simulink model "Quadcopter_2D_Control"  (R2025a)
settings: Solver=VariableStepAuto  StartTime=0.0  StopTime=10.0  RelTol=1e-3
libraries: slpidlib x3
settings Model: Creator=TAKSH MEHTA  LastModifiedBy=TAKSH MEHTA

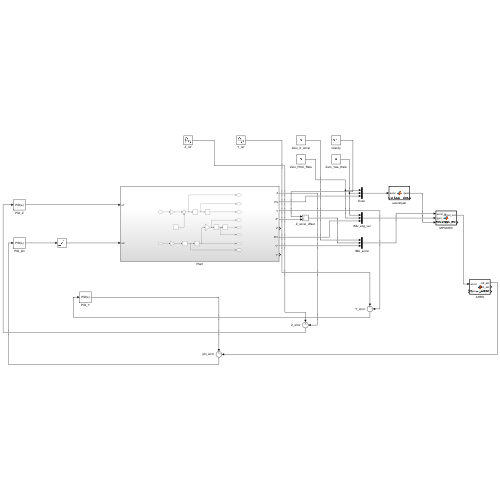
[thumbnail: Simulink's stored preview of the top-level diagram]
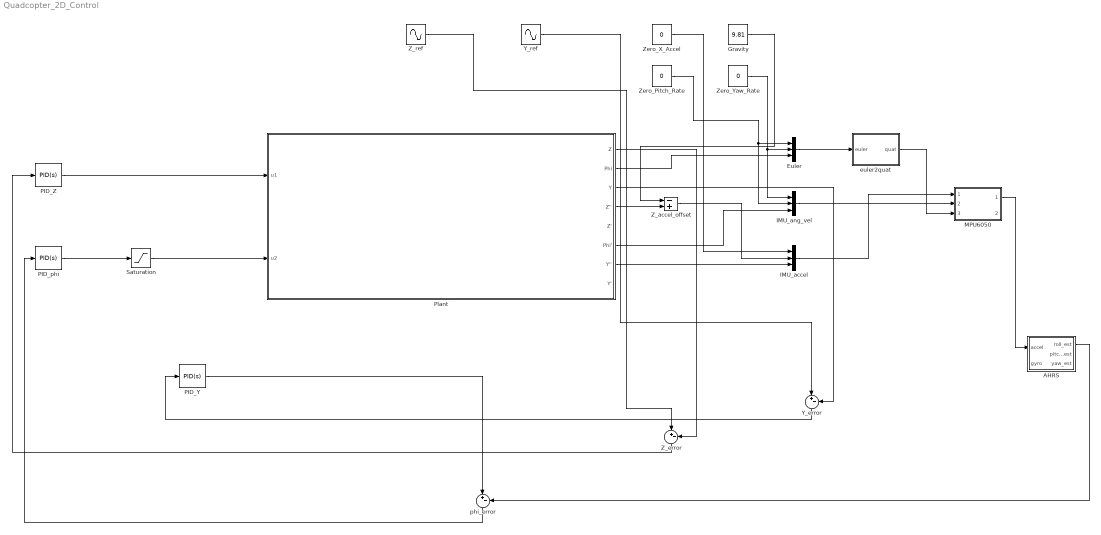
== system Quadcopter_2D_Control ==
  AHRS : MATLAB Function  TreatAsAtomicUnit=on
  Euler : Mux  Inputs=3
  Gravity : Constant  Value=9.81
  IMU_accel : Mux  Inputs=3
  IMU_ang_vel : Mux  Inputs=3
  MPU6050 : MATLAB Function  TreatAsAtomicUnit=on
  PID_Y : slpidlib/PID Controller  Controller=PID  Form=Parallel  TimeDomain=Continuous-time  UseExternalTs=off  SampleTime=-1  IntegratorMethod=Forward Euler  FilterMethod=Forward Euler  ControllerParametersSource=internal  P=2.2  I=0  UseKiTs=off  D=10  UseExternalDerivativeSource=off  N=100  UseFilter=on  TunerSelectOption=Transfer Function Based (PID Tuner App)  InitialConditionSource=internal  InitialConditionForIntegrator=0  InitialConditionForFilter=0  DifferentiatorICPrevScaledInput=0  ExternalReset=none  TrackingMode=off  Kt=1  LimitOutput=off  SatLimitsSource=internal  UpperSaturationLimit=inf  LowerSaturationLimit=-inf  LinearizeAsGain=on  AntiWindupMode=none  Kb=1  LimitIntegrator=off  UpperIntegratorSaturationLimit=inf  LowerIntegratorSaturationLimit=-inf  POutMin=[]  POutMax=[]  IOutMin=[]  IOutMax=[]  DOutMin=[]  DOutMax=[]  NOutMin=[]  NOutMax=[]  SumOutMin=[]  SumOutMax=[]  SaturationOutMin=[]  SaturationOutMax=[]  PParamMin=[]  PParamMax=[]  IParamMin=[]  IParamMax=[]  DParamMin=[]  DParamMax=[]  NParamMin=[]  NParamMax=[]  KbParamMin=[]  KbParamMax=[]  KtParamMin=[]  KtParamMax=[]  KbOutMin=[]  KbOutMax=[]  KtOutMin=[]  KtOutMax=[]  IntegratorOutMin=[]  IntegratorOutMax=[]  FilterOutMin=[]  FilterOutMax=[]  SumI1OutMin=[]  SumI1OutMax=[]  SumI2OutMin=[]  SumI2OutMax=[]  SumI3OutMin=[]  SumI3OutMax=[]  SumI4OutMin=[]  SumI4OutMax=[]  SumDOutMin=[]  SumDOutMax=[]  DifferentiatorOutMin=[]  DifferentiatorOutMax=[]  FilterDiffOutCoefMin=[]  FilterDiffOutCoefMax=[]  ReciprocalOutMin=[]  ReciprocalOutMax=[]  SumDenOutMin=[]  SumDenOutMax=[]  SumNumOutMin=[]  SumNumOutMax=[]  DivideOutMin=[]  DivideOutMax=[]  UdiffTsProdOutMin=[]  UdiffTsProdOutMax=[]  NTsProdOutMin=[]  NTsProdOutMax=[]  UintegralTsProdOutMin=[]  UintegralTsProdOutMax=[]  UngainTsProdOutMin=[]  UngainTsProdOutMax=[]  ClampingZeroOutDataTypeStr=Inherit: Inherit via back propagation  ClampingZeroOutMin=[]  ClampingZeroOutMax=[]  FilterDenConstantOutDataTypeStr=Inherit: Inherit via back propagation  FilterDenConstantOutMin=[]  FilterDenConstantOutMax=[]  PCopyOutDataTypeStr=Inherit: Inherit via back propagation  PCopyOutMin=[]  PCopyOutMax=[]  NCopyOutDataTypeStr=Inherit: Inherit via back propagation  NCopyOutMin=[]  NCopyOutMax=[]  IntegratorContinuousStateAttributes=''  IntegratorStateMustResolveToSignalObject=off  IntegratorRTWStateStorageClass=Auto  FilterContinuousStateAttributes=''  FilterStateMustResolveToSignalObject=off  FilterRTWStateStorageClass=Auto  ParallelPVariant=InternalParameters  IdealPVariant=Disabled  IVariant=InternalParameters  DVariant=InternalParameters  IntegratorVariant=Continuous  SatVariant=Disabled  AWVariant=Passthrough  PCopyVariant=Disabled  TRVariant=Disabled  FdbkBlocksVariant=Forward  IdealPFdbkVariant=Disabled  SatFdbkVariant=Disabled  DerivativeFilterVariant=ContFilter  NVariant=InternalParameters  NCopyVariant=Disabled  FilterICVariant=InternalICsFilter  IntegratorICVariant=InternalICs  ExternalResetVariant=Disabled  TRSumVariant=Passthrough  SumFdbkVariant=Disabled  SumVariant=Sum_PID  TsampFilterVariant=InternalTs  TsampNgainVariant=Passthrough  TsampIntegralVariant=Disabled_SignalSpec  ExternalSaturationOutDataTypeStr=Inherit: Same as second input  DerivativeSourceVariant=ErrorSignal  PreIntVariant=InternalPreInt
  PID_Z : slpidlib/PID Controller  Controller=PID  Form=Parallel  TimeDomain=Continuous-time  UseExternalTs=off  SampleTime=-1  IntegratorMethod=Forward Euler  FilterMethod=Forward Euler  ControllerParametersSource=internal  P=10  I=0  UseKiTs=off  D=5  UseExternalDerivativeSource=off  N=100  UseFilter=on  TunerSelectOption=Transfer Function Based (PID Tuner App)  InitialConditionSource=internal  InitialConditionForIntegrator=0  InitialConditionForFilter=0  DifferentiatorICPrevScaledInput=0  ExternalReset=none  TrackingMode=off  Kt=1  LimitOutput=off  SatLimitsSource=internal  UpperSaturationLimit=inf  LowerSaturationLimit=-inf  LinearizeAsGain=on  AntiWindupMode=none  Kb=1  LimitIntegrator=off  UpperIntegratorSaturationLimit=inf  LowerIntegratorSaturationLimit=-inf  POutMin=[]  POutMax=[]  IOutMin=[]  IOutMax=[]  DOutMin=[]  DOutMax=[]  NOutMin=[]  NOutMax=[]  SumOutMin=[]  SumOutMax=[]  SaturationOutMin=[]  SaturationOutMax=[]  PParamMin=[]  PParamMax=[]  IParamMin=[]  IParamMax=[]  DParamMin=[]  DParamMax=[]  NParamMin=[]  NParamMax=[]  KbParamMin=[]  KbParamMax=[]  KtParamMin=[]  KtParamMax=[]  KbOutMin=[]  KbOutMax=[]  KtOutMin=[]  KtOutMax=[]  IntegratorOutMin=[]  IntegratorOutMax=[]  FilterOutMin=[]  FilterOutMax=[]  SumI1OutMin=[]  SumI1OutMax=[]  SumI2OutMin=[]  SumI2OutMax=[]  SumI3OutMin=[]  SumI3OutMax=[]  SumI4OutMin=[]  SumI4OutMax=[]  SumDOutMin=[]  SumDOutMax=[]  DifferentiatorOutMin=[]  DifferentiatorOutMax=[]  FilterDiffOutCoefMin=[]  FilterDiffOutCoefMax=[]  ReciprocalOutMin=[]  ReciprocalOutMax=[]  SumDenOutMin=[]  SumDenOutMax=[]  SumNumOutMin=[]  SumNumOutMax=[]  DivideOutMin=[]  DivideOutMax=[]  UdiffTsProdOutMin=[]  UdiffTsProdOutMax=[]  NTsProdOutMin=[]  NTsProdOutMax=[]  UintegralTsProdOutMin=[]  UintegralTsProdOutMax=[]  UngainTsProdOutMin=[]  UngainTsProdOutMax=[]  ClampingZeroOutDataTypeStr=Inherit: Inherit via back propagation  ClampingZeroOutMin=[]  ClampingZeroOutMax=[]  FilterDenConstantOutDataTypeStr=Inherit: Inherit via back propagation  FilterDenConstantOutMin=[]  FilterDenConstantOutMax=[]  PCopyOutDataTypeStr=Inherit: Inherit via back propagation  PCopyOutMin=[]  PCopyOutMax=[]  NCopyOutDataTypeStr=Inherit: Inherit via back propagation  NCopyOutMin=[]  NCopyOutMax=[]  IntegratorContinuousStateAttributes=''  IntegratorStateMustResolveToSignalObject=off  IntegratorRTWStateStorageClass=Auto  FilterContinuousStateAttributes=''  FilterStateMustResolveToSignalObject=off  FilterRTWStateStorageClass=Auto  ParallelPVariant=InternalParameters  IdealPVariant=Disabled  IVariant=InternalParameters  DVariant=InternalParameters  IntegratorVariant=Continuous  SatVariant=Disabled  AWVariant=Passthrough  PCopyVariant=Disabled  TRVariant=Disabled  FdbkBlocksVariant=Forward  IdealPFdbkVariant=Disabled  SatFdbkVariant=Disabled  DerivativeFilterVariant=ContFilter  NVariant=InternalParameters  NCopyVariant=Disabled  FilterICVariant=InternalICsFilter  IntegratorICVariant=InternalICs  ExternalResetVariant=Disabled  TRSumVariant=Passthrough  SumFdbkVariant=Disabled  SumVariant=Sum_PID  TsampFilterVariant=InternalTs  TsampNgainVariant=Passthrough  TsampIntegralVariant=Disabled_SignalSpec  ExternalSaturationOutDataTypeStr=Inherit: Same as second input  DerivativeSourceVariant=ErrorSignal  PreIntVariant=InternalPreInt
  PID_phi : slpidlib/PID Controller  Controller=PID  Form=Parallel  TimeDomain=Continuous-time  UseExternalTs=off  SampleTime=-1  IntegratorMethod=Forward Euler  FilterMethod=Forward Euler  ControllerParametersSource=internal  P=50  I=0  UseKiTs=off  D=15  UseExternalDerivativeSource=off  N=100  UseFilter=on  TunerSelectOption=Transfer Function Based (PID Tuner App)  InitialConditionSource=internal  InitialConditionForIntegrator=0  InitialConditionForFilter=0  DifferentiatorICPrevScaledInput=0  ExternalReset=none  TrackingMode=off  Kt=1  LimitOutput=off  SatLimitsSource=internal  UpperSaturationLimit=inf  LowerSaturationLimit=-inf  LinearizeAsGain=on  AntiWindupMode=none  Kb=1  LimitIntegrator=off  UpperIntegratorSaturationLimit=inf  LowerIntegratorSaturationLimit=-inf  POutMin=[]  POutMax=[]  IOutMin=[]  IOutMax=[]  DOutMin=[]  DOutMax=[]  NOutMin=[]  NOutMax=[]  SumOutMin=[]  SumOutMax=[]  SaturationOutMin=[]  SaturationOutMax=[]  PParamMin=[]  PParamMax=[]  IParamMin=[]  IParamMax=[]  DParamMin=[]  DParamMax=[]  NParamMin=[]  NParamMax=[]  KbParamMin=[]  KbParamMax=[]  KtParamMin=[]  KtParamMax=[]  KbOutMin=[]  KbOutMax=[]  KtOutMin=[]  KtOutMax=[]  IntegratorOutMin=[]  IntegratorOutMax=[]  FilterOutMin=[]  FilterOutMax=[]  SumI1OutMin=[]  SumI1OutMax=[]  SumI2OutMin=[]  SumI2OutMax=[]  SumI3OutMin=[]  SumI3OutMax=[]  SumI4OutMin=[]  SumI4OutMax=[]  SumDOutMin=[]  SumDOutMax=[]  DifferentiatorOutMin=[]  DifferentiatorOutMax=[]  FilterDiffOutCoefMin=[]  FilterDiffOutCoefMax=[]  ReciprocalOutMin=[]  ReciprocalOutMax=[]  SumDenOutMin=[]  SumDenOutMax=[]  SumNumOutMin=[]  SumNumOutMax=[]  DivideOutMin=[]  DivideOutMax=[]  UdiffTsProdOutMin=[]  UdiffTsProdOutMax=[]  NTsProdOutMin=[]  NTsProdOutMax=[]  UintegralTsProdOutMin=[]  UintegralTsProdOutMax=[]  UngainTsProdOutMin=[]  UngainTsProdOutMax=[]  ClampingZeroOutDataTypeStr=Inherit: Inherit via back propagation  ClampingZeroOutMin=[]  ClampingZeroOutMax=[]  FilterDenConstantOutDataTypeStr=Inherit: Inherit via back propagation  FilterDenConstantOutMin=[]  FilterDenConstantOutMax=[]  PCopyOutDataTypeStr=Inherit: Inherit via back propagation  PCopyOutMin=[]  PCopyOutMax=[]  NCopyOutDataTypeStr=Inherit: Inherit via back propagation  NCopyOutMin=[]  NCopyOutMax=[]  IntegratorContinuousStateAttributes=''  IntegratorStateMustResolveToSignalObject=off  IntegratorRTWStateStorageClass=Auto  FilterContinuousStateAttributes=''  FilterStateMustResolveToSignalObject=off  FilterRTWStateStorageClass=Auto  ParallelPVariant=InternalParameters  IdealPVariant=Disabled  IVariant=InternalParameters  DVariant=InternalParameters  IntegratorVariant=Continuous  SatVariant=Disabled  AWVariant=Passthrough  PCopyVariant=Disabled  TRVariant=Disabled  FdbkBlocksVariant=Forward  IdealPFdbkVariant=Disabled  SatFdbkVariant=Disabled  DerivativeFilterVariant=ContFilter  NVariant=InternalParameters  NCopyVariant=Disabled  FilterICVariant=InternalICsFilter  IntegratorICVariant=InternalICs  ExternalResetVariant=Disabled  TRSumVariant=Passthrough  SumFdbkVariant=Disabled  SumVariant=Sum_PID  TsampFilterVariant=InternalTs  TsampNgainVariant=Passthrough  TsampIntegralVariant=Disabled_SignalSpec  ExternalSaturationOutDataTypeStr=Inherit: Same as second input  DerivativeSourceVariant=ErrorSignal  PreIntVariant=InternalPreInt
  Plant : Subsystem
  Saturation : Saturate  UpperLimit=0.8  LowerLimit=-0.8
  Y_error : Sum  Inputs=|+-
  Y_ref : Sin  Amplitude=0.5  Frequency=0.5  SampleTime=0
  Z_accel_offset : Sum  Inputs=-+
  Z_error : Sum  Inputs=|+-
  Z_ref : Sin  Amplitude=5  SampleTime=0
  Zero_Pitch_Rate : Constant  Value=0
  Zero_X_Accel : Constant  Value=0  OutDataTypeStr=double
  Zero_Yaw_Rate : Constant  Value=0
  euler2quat : MATLAB Function  TreatAsAtomicUnit=on
  phi_error : Sum  Inputs=|+-
  wires:
  Plant/4(Z'') -> Z_accel_offset/2
  Gravity/1 -> Z_accel_offset/1
  Plant/7(Y'') -> IMU_accel/3
  Z_accel_offset/1 -> IMU_accel/2
  Zero_X_Accel/1 -> IMU_accel/1
  Plant/6(Phi') -> IMU_ang_vel/3
  Zero_Pitch_Rate/1 -> Euler/1, IMU_ang_vel/2
  Zero_Yaw_Rate/1 -> IMU_ang_vel/1, Euler/2
  Plant/2(Phi) -> Euler/3
  Euler/1 -> euler2quat/1(euler)
  euler2quat/1(quat) -> MPU6050/3(orientation)
  IMU_accel/1 -> MPU6050/1(accel_in)
  IMU_ang_vel/1 -> MPU6050/2(gyro_in)
  MPU6050/1(accel_out) -> AHRS/1(accel)
  Plant/1(Z) -> Z_error/2
  Plant/3(Y) -> Y_error/2
  AHRS/1(roll_est) -> phi_error/2
  Z_ref/1 -> Z_error/1
  Y_ref/1 -> Y_error/1
  Z_error/1 -> PID_Z/1
  Y_error/1 -> PID_Y/1
  phi_error/1 -> PID_phi/1
  PID_Z/1 -> Plant/1(u1)
  PID_phi/1 -> Saturation/1
  Saturation/1 -> Plant/2(u2)
  PID_Y/1 -> phi_error/1

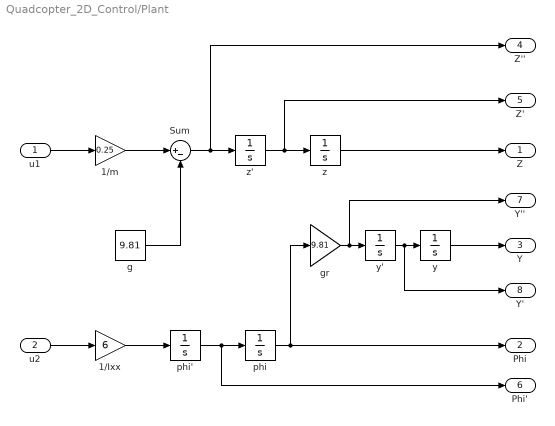
== system Quadcopter_2D_Control/Plant ==
  u1 : Inport
  u2 : Inport  Port=2
  1/Ixx : Gain  Gain=6
  1/m : Gain  Gain=0.25
  Sum : Sum  Inputs=|+-
  g : Constant  Value=9.81
  gr : Gain  Gain=9.81
  phi : Integrator
  phi' : Integrator
  y : Integrator
  y' : Integrator
  z : Integrator
  z' : Integrator
  Z : Outport
  Phi : Outport  Port=2
  Y : Outport  Port=3
  Z'' : Outport  Port=4
  Z' : Outport  Port=5
  Phi' : Outport  Port=6
  Y'' : Outport  Port=7
  Y' : Outport  Port=8
  wires:
  phi'/1 -> Phi'/1, phi/1
  u1/1 -> 1/m/1
  y'/1 -> Y'/1, y/1
  z'/1 -> Z'/1, z/1
  gr/1 -> Y''/1, y'/1
  Sum/1 -> Z''/1, z'/1
  g/1 -> Sum/2
  1/Ixx/1 -> phi'/1
  phi/1 -> Phi/1, gr/1
  u2/1 -> 1/Ixx/1
  1/m/1 -> Sum/1
  z/1 -> Z/1
  y/1 -> Y/1

== matlab function Quadcopter_2D_Control/MPU6050 ==
  data: accel_in input; accel_out output; gyro_in input; orientation input; gyro_out output
function [accel_out, gyro_out] = MPU6050_IMU(accel_in, gyro_in, orientation)
% MPU6050 IMU Sensor Model
% Inputs: accel_in [3x1], gyro_in [3x1], orientation [4x1]
% Outputs: accel_out [3x1], gyro_out [3x1] with noise

persistent accel_bias gyro_bias

% Initialize biases on first run
if isempty(accel_bias)
    accel_bias = [0.196; 0.196; 0.196];  % Constant bias (m/s²)
    gyro_bias = [0.017; 0.017; 0.017];   % Constant bias (rad/s)
end

% MPU6050 Accelerometer Parameters
accel_noise_std = 0.004 * sqrt(100);  % Noise (m/s²)
accel_noise = accel_noise_std * randn(3,1);

% MPU6050 Gyroscope Parameters
gyro_noise_std = 8.7e-5 * sqrt(100);  % Noise (rad/s)
gyro_noise = gyro_noise_std * randn(3,1);

% Add noise and bias to sensor measurements
accel_out = accel_in + accel_bias + accel_noise;
gyro_out = gyro_in + gyro_bias + gyro_noise;

end

== matlab function Quadcopter_2D_Control/euler2quat ==
  data: euler input; quat output
function quat = euler2quat_simple(euler)
    roll = euler(1); pitch = euler(2); yaw = euler(3);
    quat = [cos(roll/2)*cos(pitch/2)*cos(yaw/2) + sin(roll/2)*sin(pitch/2)*sin(yaw/2);
            sin(roll/2)*cos(pitch/2)*cos(yaw/2) - cos(roll/2)*sin(pitch/2)*sin(yaw/2);
            cos(roll/2)*sin(pitch/2)*cos(yaw/2) + sin(roll/2)*cos(pitch/2)*sin(yaw/2);
            cos(roll/2)*cos(pitch/2)*sin(yaw/2) - sin(roll/2)*sin(pitch/2)*cos(yaw/2)];
end

== matlab function Quadcopter_2D_Control/AHRS ==
  data: accel input; roll_est output; gyro input; pitch_est output; yaw_est output
function [roll_est, pitch_est, yaw_est] = Simple_AHRS(accel, gyro)
% Simple Complementary Filter for Attitude Estimation
% Inputs: accel [3x1], gyro [3x1] (rad/s)
% Outputs: roll_est, pitch_est, yaw_est (radians)

persistent roll_int pitch_int yaw_int
persistent first_run

% Filter parameters
dt = 0.01;          % Sample time (100 Hz)
alpha = 0.02;       % Complementary filter weight (2% accel, 98% gyro)

% Initialize on first run
if isempty(first_run)
    first_run = false;
    roll_int = 0;
    pitch_int = 0;
    yaw_int = 0;
end

% Extract accelerometer components
ax = accel(1); ay = accel(2); az = accel(3);

% Extract gyroscope components
gx = gyro(1); gy = gyro(2); gz = gyro(3);

% Calculate roll and pitch from accelerometer
accel_roll = atan2(ay, az);
accel_pitch = atan2(-ax, sqrt(ay^2 + az^2));

% Integrate gyroscope rates
roll_int = roll_int + gx * dt;
pitch_int = pitch_int + gy * dt;
yaw_int = yaw_int + gz * dt;

% Complementary filter (combine gyro integration with accel correction)
roll_est = alpha * accel_roll + (1 - alpha) * roll_int;
pitch_est = alpha * accel_pitch + (1 - alpha) * pitch_int;
yaw_est = yaw_int;  % No magnetometer, so just integrate gyro

% Update integrated values with filtered estimates
roll_int = roll_est;
pitch_int = pitch_est;

end
